simulink model "Relay_Auto_Tuning"  (R2017a)
settings: Solver=FixedStepAuto  StartTime=t_start  StopTime=t_end  FixedStep=dt  MaxStep=1e-1  MinStep=1e-2  RelTol=1e-3
values from neighbouring files (symbols this model uses):
  d1 = 1.4*abs(dcgain(G))    [Relay_Identification.m]
  Den = [(60-10)^(1/order)*rand+10,1]    [rtf.m]
  h = abs(min(d1,d2))*abs(dcgain(G))/mu    [Relay_Identification.m]
  L = TF.OutputDelay    [AMIGO_Detune.m]    (also in AMIGO_Tune.m = 0.2*T; Decoupling_A.m = max(L1,L2); FOTD_AREA.m = Tar-T; Relay_Identification.m = T* (tau/(1-tau)))
  Num = 1.2    [rtf.m]
  uoff = -d2*sign(dcgain(G))    [Relay_Identification.m]
  uon = d1*sign(dcgain(G))    [Relay_Identification.m]
  y0 = 0.5*max(d1,d2)    [Relay_Identification.m]
settings Model: Creator=juliu  LastModifiedBy=juliu

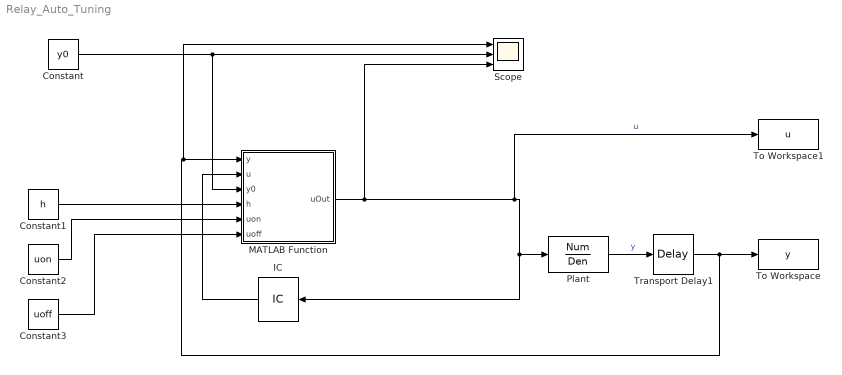
== system Relay_Auto_Tuning ==
  Constant : Constant  Value=y0
  Constant1 : Constant  Value=h
  Constant2 : Constant  Value=uon
  Constant3 : Constant  Value=uoff
  IC : InitialCondition  Value=d1
  MATLAB Function : MATLAB Function  TreatAsAtomicUnit=on
  Plant : TransferFcn  Numerator=Num  Denominator=Den
  Scope : Scope  NumInputPorts=3
  To Workspace : ToWorkspace  VariableName=y  SaveFormat=Timeseries  SampleTime=-1
  To Workspace1 : ToWorkspace  VariableName=u  SaveFormat=Timeseries  SampleTime=-1
  Transport Delay1 : TransportDelay  DelayTime=L  InitialOutput=y0  BufferSize=4096  TransDelayFeedthrough=on  PadeOrder=4
  wires:
  MATLAB Function/1(uOut) -> Scope/3, To Workspace1/1, Plant/1, IC/1  "u"
  Plant/1 -> Transport Delay1/1  "y"
  Transport Delay1/1 -> To Workspace/1, Scope/1, MATLAB Function/1(y)
  IC/1 -> MATLAB Function/2(u)
  Constant/1 -> Scope/2, MATLAB Function/3(y0)
  Constant1/1 -> MATLAB Function/4(h)
  Constant2/1 -> MATLAB Function/5(uon)
  Constant3/1 -> MATLAB Function/6(uoff)

== matlab function Relay_Auto_Tuning/MATLAB Function ==
  data: y input; u input; uOut output; y0 input; h input; uon input; uoff input
function uOut = fcn(y,u,y0,h,uon,uoff)
if y < y0-h
    uOut = uon;
elseif (y <y0+h)&&(u == uon)
    uOut = u;
elseif (y > y0-h) && (u==(uoff))
    uOut = u;
else
    uOut = uoff;
end
